simulink model "test_ffts"  (Simulink 6.2)
settings: Solver=ode45  StartTime=0.0  StopTime=300  RelTol=1e-3
undefined symbols (not defined in the file or in its folder): now
libraries: xbsIndex_r3 x1135, fft_library x1, simulink x1
(part 9 of 15)

== system test_ffts/r4_dit_fft/r4_dit_stage_3/quadplex_commutator ==
  a : Inport  Port=1  LatchInput=off
  b : Inport  Port=2  LatchInput=off
  c : Inport  Port=3  LatchInput=off
  d : Inport  Port=4  LatchInput=off
  sync_in : Inport  Port=5  LatchInput=off
  Terminator : Terminator
  biplex_commutator_01 : Subsystem  mask(Biplex Commutator){log2_size=1, n_bits=12, use_bram=off}
      mask prompts: log2_size "Log2 Block Size"; n_bits "Bit Width"; use_bram "Use BRAM"
      mask help: The biplex commutator commutes the first half of the BloBhi input "block" with the last half of the AloAhi input "block". A "block" is 2^log2_size consecutive samples (i.e. always a power of 2). sync_in precedes the first data input sample by one clock cycle. Overall latency from sync_in to sync_out is 2^(log2_size-1)+1.
      settings: AttributesFormatString=|
      | size = 2
      | delay slr
      mask Help:
      | <pre>
      | Description::
      | 
      | The biplex commutator commutes the first half of the BloBhi input "block"  with the last half
      | of the AloAhi input "block".  A "block" is 2^log2_size consecutive samples (i.e. always a
      | power of 2).
      | 
      | sync_in precedes the first data input sample by one clock cycle.
      | sync_out precedes the corresponding output sample by one clock cycle.
      | Overall latency from sync_in to sync_out is 2^(N-1)+1.
      | 
      | Mask Parameters::
      | 
      | Log 2 Block Size (log2_size): The base-2 logarithm of the length of one complete input block.
      | This MUST be an integer because the current implementation requires that
      | the input block size MUST be a power of 2.  (aka "N")
      | 
      | Bit Width (n_bits): Specifies the width of the real/imaginary components.
      | Width of each component is assumed equal.
      | 
      | Use BRAM (use_bram): Check this checkbox to implement the internal delays using BRAM.
      | If unchecked, the internal delays will be implemented using SLR16 elements.
      | </pre>
  biplex_commutator_23 : Subsystem  mask(Biplex Commutator){log2_size=1, n_bits=12, use_bram=off}
      mask prompts: log2_size "Log2 Block Size"; n_bits "Bit Width"; use_bram "Use BRAM"
      mask help: The biplex commutator commutes the first half of the BloBhi input "block" with the last half of the AloAhi input "block". A "block" is 2^log2_size consecutive samples (i.e. always a power of 2). sync_in precedes the first data input sample by one clock cycle. Overall latency from sync_in to sync_out is 2^(log2_size-1)+1.
      settings: AttributesFormatString=|
      | size = 2
      | delay slr
      mask Help:
      | <pre>
      | Description::
      | 
      | The biplex commutator commutes the first half of the BloBhi input "block"  with the last half
      | of the AloAhi input "block".  A "block" is 2^log2_size consecutive samples (i.e. always a
      | power of 2).
      | 
      | sync_in precedes the first data input sample by one clock cycle.
      | sync_out precedes the corresponding output sample by one clock cycle.
      | Overall latency from sync_in to sync_out is 2^(N-1)+1.
      | 
      | Mask Parameters::
      | 
      | Log 2 Block Size (log2_size): The base-2 logarithm of the length of one complete input block.
      | This MUST be an integer because the current implementation requires that
      | the input block size MUST be a power of 2.  (aka "N")
      | 
      | Bit Width (n_bits): Specifies the width of the real/imaginary components.
      | Width of each component is assumed equal.
      | 
      | Use BRAM (use_bram): Check this checkbox to implement the internal delays using BRAM.
      | If unchecked, the internal delays will be implemented using SLR16 elements.
      | </pre>
  biplex_commutator_ac : Subsystem  mask(Biplex Commutator){log2_size=2, n_bits=12, use_bram=off}
      mask prompts: log2_size "Log2 Block Size"; n_bits "Bit Width"; use_bram "Use BRAM"
      mask help: The biplex commutator commutes the first half of the BloBhi input "block" with the last half of the AloAhi input "block". A "block" is 2^log2_size consecutive samples (i.e. always a power of 2). sync_in precedes the first data input sample by one clock cycle. Overall latency from sync_in to sync_out is 2^(log2_size-1)+1.
      settings: AttributesFormatString=|
      | size = 4
      | delay slr
      mask Help:
      | <pre>
      | Description::
      | 
      | The biplex commutator commutes the first half of the BloBhi input "block"  with the last half
      | of the AloAhi input "block".  A "block" is 2^log2_size consecutive samples (i.e. always a
      | power of 2).
      | 
      | sync_in precedes the first data input sample by one clock cycle.
      | sync_out precedes the corresponding output sample by one clock cycle.
      | Overall latency from sync_in to sync_out is 2^(N-1)+1.
      | 
      | Mask Parameters::
      | 
      | Log 2 Block Size (log2_size): The base-2 logarithm of the length of one complete input block.
      | This MUST be an integer because the current implementation requires that
      | the input block size MUST be a power of 2.  (aka "N")
      | 
      | Bit Width (n_bits): Specifies the width of the real/imaginary components.
      | Width of each component is assumed equal.
      | 
      | Use BRAM (use_bram): Check this checkbox to implement the internal delays using BRAM.
      | If unchecked, the internal delays will be implemented using SLR16 elements.
      | </pre>
  biplex_commutator_bd : Subsystem  mask(Biplex Commutator){log2_size=2, n_bits=12, use_bram=off}
      mask prompts: log2_size "Log2 Block Size"; n_bits "Bit Width"; use_bram "Use BRAM"
      mask help: The biplex commutator commutes the first half of the BloBhi input "block" with the last half of the AloAhi input "block". A "block" is 2^log2_size consecutive samples (i.e. always a power of 2). sync_in precedes the first data input sample by one clock cycle. Overall latency from sync_in to sync_out is 2^(log2_size-1)+1.
      settings: AttributesFormatString=|
      | size = 4
      | delay slr
      mask Help:
      | <pre>
      | Description::
      | 
      | The biplex commutator commutes the first half of the BloBhi input "block"  with the last half
      | of the AloAhi input "block".  A "block" is 2^log2_size consecutive samples (i.e. always a
      | power of 2).
      | 
      | sync_in precedes the first data input sample by one clock cycle.
      | sync_out precedes the corresponding output sample by one clock cycle.
      | Overall latency from sync_in to sync_out is 2^(N-1)+1.
      | 
      | Mask Parameters::
      | 
      | Log 2 Block Size (log2_size): The base-2 logarithm of the length of one complete input block.
      | This MUST be an integer because the current implementation requires that
      | the input block size MUST be a power of 2.  (aka "N")
      | 
      | Bit Width (n_bits): Specifies the width of the real/imaginary components.
      | Width of each component is assumed equal.
      | 
      | Use BRAM (use_bram): Check this checkbox to implement the internal delays using BRAM.
      | If unchecked, the internal delays will be implemented using SLR16 elements.
      | </pre>
  abcd0 : Outport
  abcd1 : Outport  Port=2
  abcd2 : Outport  Port=3
  abcd3 : Outport  Port=4
  sync_out : Outport  Port=5
  wires:
  biplex_commutator_01/3(sync_out) -> Terminator/1
  biplex_commutator_23/3(sync_out) -> sync_out/1
  sync_in/1 -> biplex_commutator_bd/3(sync_in), biplex_commutator_ac/3(sync_in)
  d/1 -> biplex_commutator_bd/2(BloBhi)
  b/1 -> biplex_commutator_bd/1(AloAhi)
  c/1 -> biplex_commutator_ac/2(BloBhi)
  biplex_commutator_bd/3(sync_out) -> biplex_commutator_23/3(sync_in)
  biplex_commutator_bd/2(AhiBhi) -> biplex_commutator_23/2(BloBhi)
  biplex_commutator_ac/3(sync_out) -> biplex_commutator_01/3(sync_in)
  biplex_commutator_bd/1(AloBlo) -> biplex_commutator_01/2(BloBhi)
  biplex_commutator_ac/2(AhiBhi) -> biplex_commutator_23/1(AloAhi)
  biplex_commutator_23/2(AhiBhi) -> abcd3/1
  biplex_commutator_23/1(AloBlo) -> abcd2/1
  biplex_commutator_01/2(AhiBhi) -> abcd1/1
  biplex_commutator_01/1(AloBlo) -> abcd0/1
  a/1 -> biplex_commutator_ac/1(AloAhi)
  biplex_commutator_ac/1(AloBlo) -> biplex_commutator_01/1(AloAhi)

== system test_ffts/r4_dit_fft/r4_dit_stage_3/r4_butterfly ==
  a_in : Inport  Port=1  LatchInput=off
  b_in : Inport  Port=2  LatchInput=off
  c_in : Inport  Port=3  LatchInput=off
  d_in : Inport  Port=4  LatchInput=off
  sync_in : Inport  Port=5  LatchInput=off
  Terminator : Terminator
  butterfly0 : Subsystem  mask(Radix-2 Butterfly){n_bits=12, shift=0, quantization=Truncate, add_latency=1}
      mask prompts: n_bits "Bit Width In"; shift "Shift Bits"; add_latency "Adder Latency"
      mask help: The radix-2 butterfly produces a+b and a-b outputs for a and b inputs.
      settings: AttributesFormatString=shift 0
      mask Help:
      | <pre>
      | Description::
      | 
      | The radix-2 butterfly produces a+b and a-b outputs for a and b inputs.
      | The outputs are one bit wider than the inputs.
      | The output precision (i.e. the number of fractional bits) stays the same.
      | 
      | Mask Parameters::
      | 
      | Bit Width In (n_bits): Specifies the width of the real/imaginary components.
      | Width of each component is assumed equal.
      | 
      | Shift Bits (shift): Specifies how many bits to shift (down) by.  A positive value causes
      | the specified number of least significant bits to be dropped.  Usually zero or positive values
      | are used to permit or limit bit growth, but negative values can be used to induce bit growth.
      | 
      | Quantization (quantization): Specifies quantization handling (when shift bits > 0).
      | 
      | Adder Latency (add_latency): Latency to use for the underlying real adders.
      | </pre>
      mask StyleString: edit,edit,popup(Truncate|Round  (unbiased: +/- Inf)|Round  (unbiased: Even Values)),edit
  butterfly1 : Subsystem  mask(Radix-2 Butterfly){n_bits=12, shift=0, quantization=Truncate, add_latency=1}
      mask prompts: n_bits "Bit Width In"; shift "Shift Bits"; add_latency "Adder Latency"
      mask help: The radix-2 butterfly produces a+b and a-b outputs for a and b inputs.
      settings: AttributesFormatString=shift 0
      mask Help:
      | <pre>
      | Description::
      | 
      | The radix-2 butterfly produces a+b and a-b outputs for a and b inputs.
      | The outputs are one bit wider than the inputs.
      | The output precision (i.e. the number of fractional bits) stays the same.
      | 
      | Mask Parameters::
      | 
      | Bit Width In (n_bits): Specifies the width of the real/imaginary components.
      | Width of each component is assumed equal.
      | 
      | Shift Bits (shift): Specifies how many bits to shift (down) by.  A positive value causes
      | the specified number of least significant bits to be dropped.  Usually zero or positive values
      | are used to permit or limit bit growth, but negative values can be used to induce bit growth.
      | 
      | Quantization (quantization): Specifies quantization handling (when shift bits > 0).
      | 
      | Adder Latency (add_latency): Latency to use for the underlying real adders.
      | </pre>
      mask StyleString: edit,edit,popup(Truncate|Round  (unbiased: +/- Inf)|Round  (unbiased: Even Values)),edit
  butterfly2 : Subsystem  mask(Radix-2 Butterfly){n_bits=13, shift=0, quantization=Truncate, add_latency=1}
      mask prompts: n_bits "Bit Width In"; shift "Shift Bits"; add_latency "Adder Latency"
      mask help: The radix-2 butterfly produces a+b and a-b outputs for a and b inputs.
      settings: AttributesFormatString=shift 0
      mask Help:
      | <pre>
      | Description::
      | 
      | The radix-2 butterfly produces a+b and a-b outputs for a and b inputs.
      | The outputs are one bit wider than the inputs.
      | The output precision (i.e. the number of fractional bits) stays the same.
      | 
      | Mask Parameters::
      | 
      | Bit Width In (n_bits): Specifies the width of the real/imaginary components.
      | Width of each component is assumed equal.
      | 
      | Shift Bits (shift): Specifies how many bits to shift (down) by.  A positive value causes
      | the specified number of least significant bits to be dropped.  Usually zero or positive values
      | are used to permit or limit bit growth, but negative values can be used to induce bit growth.
      | 
      | Quantization (quantization): Specifies quantization handling (when shift bits > 0).
      | 
      | Adder Latency (add_latency): Latency to use for the underlying real adders.
      | </pre>
      mask StyleString: edit,edit,popup(Truncate|Round  (unbiased: +/- Inf)|Round  (unbiased: Even Values)),edit
  butterfly3j : Subsystem  mask(Radix-2 Butterfly with fixed -j twiddle (DIT, twiddle before butterfly)){n_bits=13, shift=0, quantization=Truncate, add_latency=1}
      mask prompts: n_bits "Bit Width In"; shift "Shift Bits"; add_latency "Adder Latency"
      mask help: The radix-2 butterfly with fixed DIT -j twiddle produces a-jb on the a+b output and a+jb on the a-b output for a and b inputs. It is intended for use within a radix-4 butterfly.
      settings: AttributesFormatString=shift 0
      mask Help:
      | <pre>
      | Description::
      | 
      | The radix-2 butterfly with fixed DIT -j twiddle produces a-jb on the a+b output
      | and a+jb on the a-b output for a and b inputs.
      | 
      | It is intended for use within a radix-4 butterfly.
      | 
      | The outputs are one bit wider than the inputs.
      | The output precision (i.e. the number of fractional bits) stays the same.
      | 
      | Mask Parameters::
      | 
      | Bit Width In (n_bits): Specifies the width of the real/imaginary components.
      | Width of each component is assumed equal.
      | 
      | Shift Bits (shift): Specifies how many bits to shift (down) by.  A positive value causes
      | the specified number of least significant bits to be dropped.  Usually zero or positive values
      | are used to permit or limit bit growth, but negative values can be used to induce bit growth.
      | 
      | Quantization (quantization): Specifies quantization handling (when shift bits > 0).
      | 
      | Adder Latency (add_latency): Latency to use for the underlying real adders.
      | </pre>
      mask StyleString: edit,edit,popup(Truncate|Round  (unbiased: +/- Inf)|Round  (unbiased: Even Values)),edit
  a_out : Outport
  b_out : Outport  Port=2
  c_out : Outport  Port=3
  d_out : Outport  Port=4
  sync_out : Outport  Port=5
  wires:
  butterfly2/3(sync_out) -> Terminator/1
  butterfly3j/3(sync_out) -> sync_out/1
  sync_in/1 -> butterfly0/3(sync_in), butterfly1/3(sync_in)
  butterfly3j/2(a-b) -> d_out/1
  butterfly3j/1(a+b) -> c_out/1
  butterfly2/2(a-b) -> b_out/1
  butterfly2/1(a+b) -> a_out/1
  b_in/1 -> butterfly1/1(a)
  d_in/1 -> butterfly1/2(b)
  c_in/1 -> butterfly0/2(b)
  a_in/1 -> butterfly0/1(a)
  butterfly1/1(a+b) -> butterfly2/2(b)
  butterfly0/2(a-b) -> butterfly3j/1(a)
  butterfly0/3(sync_out) -> butterfly2/3(sync_in)
  butterfly1/3(sync_out) -> butterfly3j/3(sync_in)
  butterfly1/2(a-b) -> butterfly3j/2(b)
  butterfly0/1(a+b) -> butterfly2/1(a)

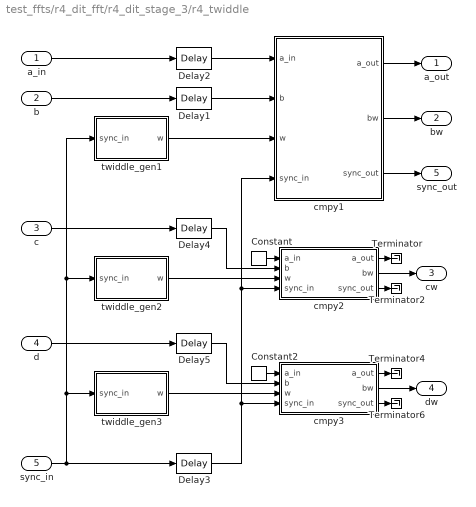
== system test_ffts/r4_dit_fft/r4_dit_stage_3/r4_twiddle ==
  a_in : Inport  Port=1  LatchInput=off
  b : Inport  Port=2  LatchInput=off
  c : Inport  Port=3  LatchInput=off
  d : Inport  Port=4  LatchInput=off
  sync_in : Inport  Port=5  LatchInput=off
  Constant : xbsIndex_r3/Constant  const=0  equ=P=C  arith_type=Unsigned  n_bits=1  bin_pt=0  opselect=C  inp2=PCIN>>17  opr=+  inp1=P  carry=CIN  iostate=0  explicit_period=on  period=1  dbl_ovrd=off
  Constant2 : xbsIndex_r3/Constant  const=0  equ=P=C  arith_type=Unsigned  n_bits=1  bin_pt=0  opselect=C  inp2=PCIN>>17  opr=+  inp1=P  carry=CIN  iostate=0  explicit_period=on  period=1  dbl_ovrd=off
  Delay{1..5} (5 alike) : xbsIndex_r3/Delay  latency=1  reg_retiming=off  explicit_period=off  period=1  en=off  accept_only_valid=off  init_zero=on  dbl_ovrd=off  show_param=off
      settings: xl_area=[0, 0, 0, 0, 0, 0, 0]
  Terminator{,2,4,6} (4 alike) : Terminator
  cmpy1 : Subsystem  mask(Complex Multiplier (4 real multipliers)){n_bits_b=12, bin_pt_b=11, n_bits_w=9, bin_pt_w=7, n_bits_bw=12, bin_pt_bw=11, quantization=Round  (unbiased: Even Values), overflow=Wrap, mult_latency=3, add_latency=1}
      mask prompts: n_bits_b "Number of Bits B"; bin_pt_b "Binary Point B"; n_bits_w "Number of Bits W"; bin_pt_w "Binary Point W"; n_bits_bw "Number of Bits BW"; bin_pt_bw "Binary Point BW"; mult_latency "Multiplier Latency"; add_latency "Adder Latency"
      mask help: This block multiplies two complex numbers using 4 real multipliers and 2 real adders. Pass-through paths are provided for another complex number and a sync signal. These pass through paths provide delay that matches the latency of the complex multiply operation.
      settings: AttributesFormatString=|
      | 12_11 * 9_7 ==> 12_11
      | round even, wrap
      | 3 mults
      mask Help:
      | <pre>
      | Description::
      | 
      | This block multiplies two complex numbers using 4 real multipliers and 2 real adders.
      | Pass-through paths are provided for another complex number and a sync signal.
      | These paths provide delay that matches the latency of the complex multiply operation.
      | 
      | a_in is passed through to a_out.
      | b and w complex inputs are multiplied and their product appears on the bw output.
      | sync_in is passed through to sync_out.
      | 
      | Mask Parameters::
      | 
      | Number of Bits B (n_bits_b): Specifies the width of the real/imaginary
      | components of input b.  Assumed equal for both components.
      | 
      | Binary Point B (bin_pt_b): Specifies the binary point point position of the
      | real/imaginary components of input b.  Assumed equal for both components.
      | 
      | Number of Bits W (n_bits_w): Specifies the width of the real/imaginary
      | components of input w.  Assumed equal for both components.
      | 
      | Binary Point W (bin_pt_w): Specifies the binary point point position of the
      | real/imaginary components of input w.  Assumed equal for both components.
      | 
      | Number of Bits BW (n_bits_bw): Specifies the width of the real/imaginary
      | components of output bw.  Assumed equal for both components.
      | 
      | Binary Point BW (bin_pt_bw): Specifies the binary point point position of the
      | real/imaginary components of output bw.  Assumed equal for both components.
      | 
      | Quantization (quantization): Specifies quantization handling.
      | 
      | Overflow (overflow): Specifies overflow handling.
      | 
      | Multiplier Latency (mult_latency): Latency to use for the underlying real multipliers.
      | 
      | Adder Latency (add_latency): Latency to use for the underlying real adders.
      | </pre>
      mask StyleString: edit,edit,edit,edit,edit,edit,popup(Truncate|Round  (unbiased: +/- Inf)|Round  (unbiased: Even Values)),popup(Wrap|Saturate|Error),edit,edit
  cmpy2 : Subsystem  mask(Complex Multiplier (4 real multipliers)){n_bits_b=12, bin_pt_b=11, n_bits_w=9, bin_pt_w=7, n_bits_bw=12, bin_pt_bw=11, quantization=Round  (unbiased: Even Values), overflow=Wrap, mult_latency=3, add_latency=1}
      mask prompts: n_bits_b "Number of Bits B"; bin_pt_b "Binary Point B"; n_bits_w "Number of Bits W"; bin_pt_w "Binary Point W"; n_bits_bw "Number of Bits BW"; bin_pt_bw "Binary Point BW"; mult_latency "Multiplier Latency"; add_latency "Adder Latency"
      mask help: This block multiplies two complex numbers using 4 real multipliers and 2 real adders. Pass-through paths are provided for another complex number and a sync signal. These pass through paths provide delay that matches the latency of the complex multiply operation.
      settings: AttributesFormatString=|
      | 12_11 * 9_7 ==> 12_11
      | round even, wrap
      | 3 mults
      mask Help:
      | <pre>
      | Description::
      | 
      | This block multiplies two complex numbers using 4 real multipliers and 2 real adders.
      | Pass-through paths are provided for another complex number and a sync signal.
      | These paths provide delay that matches the latency of the complex multiply operation.
      | 
      | a_in is passed through to a_out.
      | b and w complex inputs are multiplied and their product appears on the bw output.
      | sync_in is passed through to sync_out.
      | 
      | Mask Parameters::
      | 
      | Number of Bits B (n_bits_b): Specifies the width of the real/imaginary
      | components of input b.  Assumed equal for both components.
      | 
      | Binary Point B (bin_pt_b): Specifies the binary point point position of the
      | real/imaginary components of input b.  Assumed equal for both components.
      | 
      | Number of Bits W (n_bits_w): Specifies the width of the real/imaginary
      | components of input w.  Assumed equal for both components.
      | 
      | Binary Point W (bin_pt_w): Specifies the binary point point position of the
      | real/imaginary components of input w.  Assumed equal for both components.
      | 
      | Number of Bits BW (n_bits_bw): Specifies the width of the real/imaginary
      | components of output bw.  Assumed equal for both components.
      | 
      | Binary Point BW (bin_pt_bw): Specifies the binary point point position of the
      | real/imaginary components of output bw.  Assumed equal for both components.
      | 
      | Quantization (quantization): Specifies quantization handling.
      | 
      | Overflow (overflow): Specifies overflow handling.
      | 
      | Multiplier Latency (mult_latency): Latency to use for the underlying real multipliers.
      | 
      | Adder Latency (add_latency): Latency to use for the underlying real adders.
      | </pre>
      mask StyleString: edit,edit,edit,edit,edit,edit,popup(Truncate|Round  (unbiased: +/- Inf)|Round  (unbiased: Even Values)),popup(Wrap|Saturate|Error),edit,edit
  cmpy3 : Subsystem  mask(Complex Multiplier (4 real multipliers)){n_bits_b=12, bin_pt_b=11, n_bits_w=9, bin_pt_w=7, n_bits_bw=12, bin_pt_bw=11, quantization=Round  (unbiased: Even Values), overflow=Wrap, mult_latency=3, add_latency=1}
      mask prompts: n_bits_b "Number of Bits B"; bin_pt_b "Binary Point B"; n_bits_w "Number of Bits W"; bin_pt_w "Binary Point W"; n_bits_bw "Number of Bits BW"; bin_pt_bw "Binary Point BW"; mult_latency "Multiplier Latency"; add_latency "Adder Latency"
      mask help: This block multiplies two complex numbers using 4 real multipliers and 2 real adders. Pass-through paths are provided for another complex number and a sync signal. These pass through paths provide delay that matches the latency of the complex multiply operation.
      settings: AttributesFormatString=|
      | 12_11 * 9_7 ==> 12_11
      | round even, wrap
      | 3 mults
      mask Help:
      | <pre>
      | Description::
      | 
      | This block multiplies two complex numbers using 4 real multipliers and 2 real adders.
      | Pass-through paths are provided for another complex number and a sync signal.
      | These paths provide delay that matches the latency of the complex multiply operation.
      | 
      | a_in is passed through to a_out.
      | b and w complex inputs are multiplied and their product appears on the bw output.
      | sync_in is passed through to sync_out.
      | 
      | Mask Parameters::
      | 
      | Number of Bits B (n_bits_b): Specifies the width of the real/imaginary
      | components of input b.  Assumed equal for both components.
      | 
      | Binary Point B (bin_pt_b): Specifies the binary point point position of the
      | real/imaginary components of input b.  Assumed equal for both components.
      | 
      | Number of Bits W (n_bits_w): Specifies the width of the real/imaginary
      | components of input w.  Assumed equal for both components.
      | 
      | Binary Point W (bin_pt_w): Specifies the binary point point position of the
      | real/imaginary components of input w.  Assumed equal for both components.
      | 
      | Number of Bits BW (n_bits_bw): Specifies the width of the real/imaginary
      | components of output bw.  Assumed equal for both components.
      | 
      | Binary Point BW (bin_pt_bw): Specifies the binary point point position of the
      | real/imaginary components of output bw.  Assumed equal for both components.
      | 
      | Quantization (quantization): Specifies quantization handling.
      | 
      | Overflow (overflow): Specifies overflow handling.
      | 
      | Multiplier Latency (mult_latency): Latency to use for the underlying real multipliers.
      | 
      | Adder Latency (add_latency): Latency to use for the underlying real adders.
      | </pre>
      mask StyleString: edit,edit,edit,edit,edit,edit,popup(Truncate|Round  (unbiased: +/- Inf)|Round  (unbiased: Even Values)),popup(Wrap|Saturate|Error),edit,edit
  twiddle_gen1 : Subsystem  mask(Radix-R Twiddle Coefficient Generator (complex storage)){n_stages=3, radix=4, cur_stage=3, branch=1, decimation=Time, n_bits_w=9, bin_pt_w=7, use_bram=off}
      mask prompts: n_stages "Total Stages"; cur_stage "Current Stage"; decimation "Decimation Mode"; n_bits_w "Number of Bits"; bin_pt_w "Binary Point"; use_bram "Use BRAM"
      mask help: A radix-R twiddle coefficient generator using complex storage. Generates twiddle factors for Decimation in Time (i.e. twiddles before butterflies) or Decimation in Frequency (i.e. twiddles after butterflies) Fast Fourier Transforms of arbitrary-but-fixed radix. Radix must be a power of 2. Regardless of the decimation mode, the FFT is assumed to have inputs in normal order and outputs in bit-reversed order.
      settings: AttributesFormatString=|
      | depth 16
      | twiddle dist
      mask Help:
      | <pre>
      | Description::
      | 
      | A radix-R twiddle coefficient generator using complex storage.
      | 
      | Generates twiddle factors for Decimation in Time (i.e. twiddles before butterflies)
      | or Decimation in Frequency (i.e. twiddles after butterflies) Fast Fourier Transforms
      | of arbitrary-but-fixed radix.  Radix must be a power of 2.
      | 
      | Regardless of the decimation mode, the FFT is assumed to have inputs normally
      | ordered and outputs in bit-reversed order.
      | 
      | Complex storage means that the real and imaginary components are stored in
      | the same memory element.  This is generally fine, but if the combined width of
      | the real and imaginary components is greater than 18 and BRAM is being used
      | for the underlying storage, then the multiplier(s) adjacent to the BRAM(s) will
      | not be usable.  If that is a problem for your design, consider using the
      | "Radix-R Twiddle Coefficient Generator (real/imag storage)" block.
      | 
      | Mask Parameters::
      | 
      | Total Stages (n_stages):  The number of total stages in the FFT.
      | 
      | Radix (radix): The radix of the FFT.  The FFT will have radix^n_stages points.
      | 
      | Current Stage (cur_stage):  The number of the current stage for which this block should
      | generate twiddle coefficients.  Valid values are 3 through n_stages, inclusive.  Note that
      | stages are counted from 1 to n_stages for DIT (i.e. cur_stage==1 for the first stage) and
      | n_stages to 1 for DIF (i.e. cur_stage==1 for the last stage).
      | 
      | Branch (branch): The butterfly branch associated with this twiddle generator.
      | Valid values are 1 through radix-1, inclusive.
      | 
      | Decimation Mode (decimation): The decimation mode of the FFT.
      | 
      | Number of Bits (n_bits_w): Specifies the width of the real/imaginary components.
      | Assumed equal for both components.  This block outputs UFix_(2*n_bits_w)_0.
      | 
      | Use BRAM (use_bram): Check this checkbox to store twiddle coefficients in BRAM.
      | If unchecked, the coefficients will be sored in distributed memory (i.e. slices).
      | </pre>
      mask StyleString: edit,edit,edit,edit,popup(Time|Frequency),edit,edit,checkbox
  twiddle_gen2 : Subsystem  mask(Radix-R Twiddle Coefficient Generator (complex storage)){n_stages=3, radix=4, cur_stage=3, branch=2, decimation=Time, n_bits_w=9, bin_pt_w=7, use_bram=off}
      mask prompts: n_stages "Total Stages"; cur_stage "Current Stage"; decimation "Decimation Mode"; n_bits_w "Number of Bits"; bin_pt_w "Binary Point"; use_bram "Use BRAM"
      mask help: A radix-R twiddle coefficient generator using complex storage. Generates twiddle factors for Decimation in Time (i.e. twiddles before butterflies) or Decimation in Frequency (i.e. twiddles after butterflies) Fast Fourier Transforms of arbitrary-but-fixed radix. Radix must be a power of 2. Regardless of the decimation mode, the FFT is assumed to have inputs in normal order and outputs in bit-reversed order.
      settings: AttributesFormatString=|
      | depth 16
      | twiddle dist
      mask Help:
      | <pre>
      | Description::
      | 
      | A radix-R twiddle coefficient generator using complex storage.
      | 
      | Generates twiddle factors for Decimation in Time (i.e. twiddles before butterflies)
      | or Decimation in Frequency (i.e. twiddles after butterflies) Fast Fourier Transforms
      | of arbitrary-but-fixed radix.  Radix must be a power of 2.
      | 
      | Regardless of the decimation mode, the FFT is assumed to have inputs normally
      | ordered and outputs in bit-reversed order.
      | 
      | Complex storage means that the real and imaginary components are stored in
      | the same memory element.  This is generally fine, but if the combined width of
      | the real and imaginary components is greater than 18 and BRAM is being used
      | for the underlying storage, then the multiplier(s) adjacent to the BRAM(s) will
      | not be usable.  If that is a problem for your design, consider using the
      | "Radix-R Twiddle Coefficient Generator (real/imag storage)" block.
      | 
      | Mask Parameters::
      | 
      | Total Stages (n_stages):  The number of total stages in the FFT.
      | 
      | Radix (radix): The radix of the FFT.  The FFT will have radix^n_stages points.
      | 
      | Current Stage (cur_stage):  The number of the current stage for which this block should
      | generate twiddle coefficients.  Valid values are 3 through n_stages, inclusive.  Note that
      | stages are counted from 1 to n_stages for DIT (i.e. cur_stage==1 for the first stage) and
      | n_stages to 1 for DIF (i.e. cur_stage==1 for the last stage).
      | 
      | Branch (branch): The butterfly branch associated with this twiddle generator.
      | Valid values are 1 through radix-1, inclusive.
      | 
      | Decimation Mode (decimation): The decimation mode of the FFT.
      | 
      | Number of Bits (n_bits_w): Specifies the width of the real/imaginary components.
      | Assumed equal for both components.  This block outputs UFix_(2*n_bits_w)_0.
      | 
      | Use BRAM (use_bram): Check this checkbox to store twiddle coefficients in BRAM.
      | If unchecked, the coefficients will be sored in distributed memory (i.e. slices).
      | </pre>
      mask StyleString: edit,edit,edit,edit,popup(Time|Frequency),edit,edit,checkbox
  twiddle_gen3 : Subsystem  mask(Radix-R Twiddle Coefficient Generator (complex storage)){n_stages=3, radix=4, cur_stage=3, branch=3, decimation=Time, n_bits_w=9, bin_pt_w=7, use_bram=off}
      mask prompts: n_stages "Total Stages"; cur_stage "Current Stage"; decimation "Decimation Mode"; n_bits_w "Number of Bits"; bin_pt_w "Binary Point"; use_bram "Use BRAM"
      mask help: A radix-R twiddle coefficient generator using complex storage. Generates twiddle factors for Decimation in Time (i.e. twiddles before butterflies) or Decimation in Frequency (i.e. twiddles after butterflies) Fast Fourier Transforms of arbitrary-but-fixed radix. Radix must be a power of 2. Regardless of the decimation mode, the FFT is assumed to have inputs in normal order and outputs in bit-reversed order.
      settings: AttributesFormatString=|
      | depth 16
      | twiddle dist
      mask Help:
      | <pre>
      | Description::
      | 
      | A radix-R twiddle coefficient generator using complex storage.
      | 
      | Generates twiddle factors for Decimation in Time (i.e. twiddles before butterflies)
      | or Decimation in Frequency (i.e. twiddles after butterflies) Fast Fourier Transforms
      | of arbitrary-but-fixed radix.  Radix must be a power of 2.
      | 
      | Regardless of the decimation mode, the FFT is assumed to have inputs normally
      | ordered and outputs in bit-reversed order.
      | 
      | Complex storage means that the real and imaginary components are stored in
      | the same memory element.  This is generally fine, but if the combined width of
      | the real and imaginary components is greater than 18 and BRAM is being used
      | for the underlying storage, then the multiplier(s) adjacent to the BRAM(s) will
      | not be usable.  If that is a problem for your design, consider using the
      | "Radix-R Twiddle Coefficient Generator (real/imag storage)" block.
      | 
      | Mask Parameters::
      | 
      | Total Stages (n_stages):  The number of total stages in the FFT.
      | 
      | Radix (radix): The radix of the FFT.  The FFT will have radix^n_stages points.
      | 
      | Current Stage (cur_stage):  The number of the current stage for which this block should
      | generate twiddle coefficients.  Valid values are 3 through n_stages, inclusive.  Note that
      | stages are counted from 1 to n_stages for DIT (i.e. cur_stage==1 for the first stage) and
      | n_stages to 1 for DIF (i.e. cur_stage==1 for the last stage).
      | 
      | Branch (branch): The butterfly branch associated with this twiddle generator.
      | Valid values are 1 through radix-1, inclusive.
      | 
      | Decimation Mode (decimation): The decimation mode of the FFT.
      | 
      | Number of Bits (n_bits_w): Specifies the width of the real/imaginary components.
      | Assumed equal for both components.  This block outputs UFix_(2*n_bits_w)_0.
      | 
      | Use BRAM (use_bram): Check this checkbox to store twiddle coefficients in BRAM.
      | If unchecked, the coefficients will be sored in distributed memory (i.e. slices).
      | </pre>
      mask StyleString: edit,edit,edit,edit,popup(Time|Frequency),edit,edit,checkbox
  a_out : Outport
  bw : Outport  Port=2
  cw : Outport  Port=3
  dw : Outport  Port=4
  sync_out : Outport  Port=5
  wires:
  Delay3/1 -> cmpy2/4(sync_in), cmpy1/4(sync_in), cmpy3/4(sync_in)
  cmpy3/3(sync_out) -> Terminator6/1
  cmpy3/1(a_out) -> Terminator4/1
  Constant2/1 -> cmpy3/1(a_in)
  cmpy2/3(sync_out) -> Terminator2/1
  cmpy2/1(a_out) -> Terminator/1
  Constant/1 -> cmpy2/1(a_in)
  Delay5/1 -> cmpy3/2(b)
  d/1 -> Delay5/1
  Delay4/1 -> cmpy2/2(b)
  c/1 -> Delay4/1
  twiddle_gen3/1(w) -> cmpy3/3(w)
  twiddle_gen2/1(w) -> cmpy2/3(w)
  cmpy3/2(bw) -> dw/1
  cmpy2/2(bw) -> cw/1
  sync_in/1 -> twiddle_gen3/1(sync_in), twiddle_gen2/1(sync_in), twiddle_gen1/1(sync_in), Delay3/1
  b/1 -> Delay1/1
  a_in/1 -> Delay2/1
  Delay2/1 -> cmpy1/1(a_in)
  cmpy1/1(a_out) -> a_out/1
  Delay1/1 -> cmpy1/2(b)
  cmpy1/2(bw) -> bw/1
  twiddle_gen1/1(w) -> cmpy1/3(w)
  cmpy1/3(sync_out) -> sync_out/1

== system test_ffts/r2_dit_fft/biplex_commutator/delay_b/c_to_ri ==
  c : Inport  Port=1  LatchInput=off
  force_im : xbsIndex_r3/Reinterpret  force_arith_type=on  arith_type="Signed  (2's comp)"  force_bin_pt=on  bin_pt=0  force_valid=on
  force_re : xbsIndex_r3/Reinterpret  force_arith_type=on  arith_type="Signed  (2's comp)"  force_bin_pt=on  bin_pt=0  force_valid=on
  slice_im : xbsIndex_r3/Slice  mode=Lower Bit Location + Width  nbits=14  bit1=0  base1=MSB of Input  bit0=0  base0=LSB of Input  boolean_output=off  explicit_period=off  period=1  dbl_ovrd=off
  slice_re : xbsIndex_r3/Slice  mode=Upper Bit Location + Width  nbits=14  bit1=0  base1=MSB of Input  bit0=0  base0=LSB of Input  boolean_output=off  explicit_period=off  period=1  dbl_ovrd=off
  re : Outport
  im : Outport  Port=2
  wires:
  slice_re/1 -> force_re/1
  slice_im/1 -> force_im/1
  force_re/1 -> re/1
  force_im/1 -> im/1
  c/1 -> slice_re/1, slice_im/1

== system test_ffts/r2_dit_fft/biplex_commutator/delay_b/delay_im ==
  in : Inport  Port=1  LatchInput=off
  Constant : xbsIndex_r3/Constant  const=1  equ=P=C  arith_type=Boolean  n_bits=1  bin_pt=0  opselect=C  inp2=PCIN>>17  opr=+  inp1=P  carry=CIN  iostate=0  explicit_period=on  period=1  dbl_ovrd=off
  Counter : xbsIndex_r3/Counter  cnt_type=Count Limited  n_bits=5  bin_pt=0  arith_type=Unsigned  start_count=0  cnt_to=30  cnt_by_val=1  operation=Up  explicit_period=off  period=1  load_pin=off  rst=off  en=off  dbl_ovrd=off  show_param=off  use_rpm=on  gen_core=off
      settings: xl_area=[0, 0, 0, 0, 0, 0, 0]
  bram : xbsIndex_r3/Single Port RAM  depth=32  initVector=0  write_mode=Read Before Write  latency=1  init_zero=on  explicit_period=off  period=1  rst=off  init_reg=0  en=off  dbl_ovrd=off  show_param=off  distributed_mem=off  use_rpm=off  gen_core=off
      settings: xl_area=[0, 0, 0, 0, 0, 0, 0]
  out : Outport
  wires:
  Constant/1 -> bram/3
  in/1 -> bram/2
  bram/1 -> out/1
  Counter/1 -> bram/1

== system test_ffts/r2_dit_fft/biplex_commutator/delay_b/delay_re ==
  in : Inport  Port=1  LatchInput=off
  Constant : xbsIndex_r3/Constant  const=1  equ=P=C  arith_type=Boolean  n_bits=1  bin_pt=0  opselect=C  inp2=PCIN>>17  opr=+  inp1=P  carry=CIN  iostate=0  explicit_period=on  period=1  dbl_ovrd=off
  Counter : xbsIndex_r3/Counter  cnt_type=Count Limited  n_bits=5  bin_pt=0  arith_type=Unsigned  start_count=0  cnt_to=30  cnt_by_val=1  operation=Up  explicit_period=off  period=1  load_pin=off  rst=off  en=off  dbl_ovrd=off  show_param=off  use_rpm=on  gen_core=off
      settings: xl_area=[0, 0, 0, 0, 0, 0, 0]
  bram : xbsIndex_r3/Single Port RAM  depth=32  initVector=0  write_mode=Read Before Write  latency=1  init_zero=on  explicit_period=off  period=1  rst=off  init_reg=0  en=off  dbl_ovrd=off  show_param=off  distributed_mem=off  use_rpm=off  gen_core=off
      settings: xl_area=[0, 0, 0, 0, 0, 0, 0]
  out : Outport
  wires:
  Constant/1 -> bram/3
  in/1 -> bram/2
  bram/1 -> out/1
  Counter/1 -> bram/1

== system test_ffts/r2_dit_fft/biplex_commutator/delay_b/ri_to_c ==
  re : Inport  Port=1  LatchInput=off
  im : Inport  Port=2  LatchInput=off
  concat : xbsIndex_r3/Concat  num_inputs=2  explicit_period=off  period=1  dbl_ovrd=off
  force_im : xbsIndex_r3/Reinterpret  force_arith_type=on  arith_type=Unsigned  force_bin_pt=on  bin_pt=0  force_valid=on
  force_re : xbsIndex_r3/Reinterpret  force_arith_type=on  arith_type=Unsigned  force_bin_pt=on  bin_pt=0  force_valid=on
  c : Outport
  wires:
  force_re/1 -> concat/1
  force_im/1 -> concat/2
  re/1 -> force_re/1
  concat/1 -> c/1
  im/1 -> force_im/1

== system test_ffts/r2_dit_fft/biplex_commutator/delay_lo/c_to_ri ==
  c : Inport  Port=1  LatchInput=off
  force_im : xbsIndex_r3/Reinterpret  force_arith_type=on  arith_type="Signed  (2's comp)"  force_bin_pt=on  bin_pt=0  force_valid=on
  force_re : xbsIndex_r3/Reinterpret  force_arith_type=on  arith_type="Signed  (2's comp)"  force_bin_pt=on  bin_pt=0  force_valid=on
  slice_im : xbsIndex_r3/Slice  mode=Lower Bit Location + Width  nbits=14  bit1=0  base1=MSB of Input  bit0=0  base0=LSB of Input  boolean_output=off  explicit_period=off  period=1  dbl_ovrd=off
  slice_re : xbsIndex_r3/Slice  mode=Upper Bit Location + Width  nbits=14  bit1=0  base1=MSB of Input  bit0=0  base0=LSB of Input  boolean_output=off  explicit_period=off  period=1  dbl_ovrd=off
  re : Outport
  im : Outport  Port=2
  wires:
  slice_re/1 -> force_re/1
  slice_im/1 -> force_im/1
  force_re/1 -> re/1
  force_im/1 -> im/1
  c/1 -> slice_re/1, slice_im/1

== system test_ffts/r2_dit_fft/biplex_commutator/delay_lo/delay_im ==
  in : Inport  Port=1  LatchInput=off
  Constant : xbsIndex_r3/Constant  const=1  equ=P=C  arith_type=Boolean  n_bits=1  bin_pt=0  opselect=C  inp2=PCIN>>17  opr=+  inp1=P  carry=CIN  iostate=0  explicit_period=on  period=1  dbl_ovrd=off
  Counter : xbsIndex_r3/Counter  cnt_type=Count Limited  n_bits=5  bin_pt=0  arith_type=Unsigned  start_count=0  cnt_to=30  cnt_by_val=1  operation=Up  explicit_period=off  period=1  load_pin=off  rst=off  en=off  dbl_ovrd=off  show_param=off  use_rpm=on  gen_core=off
      settings: xl_area=[0, 0, 0, 0, 0, 0, 0]
  bram : xbsIndex_r3/Single Port RAM  depth=32  initVector=0  write_mode=Read Before Write  latency=1  init_zero=on  explicit_period=off  period=1  rst=off  init_reg=0  en=off  dbl_ovrd=off  show_param=off  distributed_mem=off  use_rpm=off  gen_core=off
      settings: xl_area=[0, 0, 0, 0, 0, 0, 0]
  out : Outport
  wires:
  Constant/1 -> bram/3
  in/1 -> bram/2
  bram/1 -> out/1
  Counter/1 -> bram/1

== system test_ffts/r2_dit_fft/biplex_commutator/delay_lo/delay_re ==
  in : Inport  Port=1  LatchInput=off
  Constant : xbsIndex_r3/Constant  const=1  equ=P=C  arith_type=Boolean  n_bits=1  bin_pt=0  opselect=C  inp2=PCIN>>17  opr=+  inp1=P  carry=CIN  iostate=0  explicit_period=on  period=1  dbl_ovrd=off
  Counter : xbsIndex_r3/Counter  cnt_type=Count Limited  n_bits=5  bin_pt=0  arith_type=Unsigned  start_count=0  cnt_to=30  cnt_by_val=1  operation=Up  explicit_period=off  period=1  load_pin=off  rst=off  en=off  dbl_ovrd=off  show_param=off  use_rpm=on  gen_core=off
      settings: xl_area=[0, 0, 0, 0, 0, 0, 0]
  bram : xbsIndex_r3/Single Port RAM  depth=32  initVector=0  write_mode=Read Before Write  latency=1  init_zero=on  explicit_period=off  period=1  rst=off  init_reg=0  en=off  dbl_ovrd=off  show_param=off  distributed_mem=off  use_rpm=off  gen_core=off
      settings: xl_area=[0, 0, 0, 0, 0, 0, 0]
  out : Outport
  wires:
  Constant/1 -> bram/3
  in/1 -> bram/2
  bram/1 -> out/1
  Counter/1 -> bram/1

== system test_ffts/r2_dit_fft/biplex_commutator/delay_lo/ri_to_c ==
  re : Inport  Port=1  LatchInput=off
  im : Inport  Port=2  LatchInput=off
  concat : xbsIndex_r3/Concat  num_inputs=2  explicit_period=off  period=1  dbl_ovrd=off
  force_im : xbsIndex_r3/Reinterpret  force_arith_type=on  arith_type=Unsigned  force_bin_pt=on  bin_pt=0  force_valid=on
  force_re : xbsIndex_r3/Reinterpret  force_arith_type=on  arith_type=Unsigned  force_bin_pt=on  bin_pt=0  force_valid=on
  c : Outport
  wires:
  force_re/1 -> concat/1
  force_im/1 -> concat/2
  re/1 -> force_re/1
  concat/1 -> c/1
  im/1 -> force_im/1

== system test_ffts/r2_dit_fft/r2_dit_stage_1/biplex_commutator/delay_b ==
  in : Inport  Port=1  LatchInput=off
  slr : xbsIndex_r3/Delay  latency=32  reg_retiming=off  explicit_period=off  period=1  en=off  accept_only_valid=off  init_zero=on  dbl_ovrd=off  show_param=off
      settings: xl_area=[0, 0, 0, 0, 0, 0, 0]
  out : Outport
  wires:
  slr/1 -> out/1
  in/1 -> slr/1

== system test_ffts/r2_dit_fft/r2_dit_stage_1/biplex_commutator/delay_lo ==
  in : Inport  Port=1  LatchInput=off
  slr : xbsIndex_r3/Delay  latency=32  reg_retiming=off  explicit_period=off  period=1  en=off  accept_only_valid=off  init_zero=on  dbl_ovrd=off  show_param=off
      settings: xl_area=[0, 0, 0, 0, 0, 0, 0]
  out : Outport
  wires:
  slr/1 -> out/1
  in/1 -> slr/1

== system test_ffts/r2_dit_fft/r2_dit_stage_1/r2_butterfly/c_to_ri ==
  c : Inport  Port=1  LatchInput=off
  force_im : xbsIndex_r3/Reinterpret  force_arith_type=on  arith_type="Signed  (2's comp)"  force_bin_pt=on  bin_pt=0  force_valid=on
  force_re : xbsIndex_r3/Reinterpret  force_arith_type=on  arith_type="Signed  (2's comp)"  force_bin_pt=on  bin_pt=0  force_valid=on
  slice_im : xbsIndex_r3/Slice  mode=Lower Bit Location + Width  nbits=8  bit1=0  base1=MSB of Input  bit0=0  base0=LSB of Input  boolean_output=off  explicit_period=off  period=1  dbl_ovrd=off
  slice_re : xbsIndex_r3/Slice  mode=Upper Bit Location + Width  nbits=8  bit1=0  base1=MSB of Input  bit0=0  base0=LSB of Input  boolean_output=off  explicit_period=off  period=1  dbl_ovrd=off
  re : Outport
  im : Outport  Port=2
  wires:
  slice_re/1 -> force_re/1
  slice_im/1 -> force_im/1
  force_re/1 -> re/1
  force_im/1 -> im/1
  c/1 -> slice_re/1, slice_im/1

== system test_ffts/r2_dit_fft/r2_dit_stage_1/r2_butterfly/c_to_ri1 ==
  c : Inport  Port=1  LatchInput=off
  force_im : xbsIndex_r3/Reinterpret  force_arith_type=on  arith_type="Signed  (2's comp)"  force_bin_pt=on  bin_pt=0  force_valid=on
  force_re : xbsIndex_r3/Reinterpret  force_arith_type=on  arith_type="Signed  (2's comp)"  force_bin_pt=on  bin_pt=0  force_valid=on
  slice_im : xbsIndex_r3/Slice  mode=Lower Bit Location + Width  nbits=8  bit1=0  base1=MSB of Input  bit0=0  base0=LSB of Input  boolean_output=off  explicit_period=off  period=1  dbl_ovrd=off
  slice_re : xbsIndex_r3/Slice  mode=Upper Bit Location + Width  nbits=8  bit1=0  base1=MSB of Input  bit0=0  base0=LSB of Input  boolean_output=off  explicit_period=off  period=1  dbl_ovrd=off
  re : Outport
  im : Outport  Port=2
  wires:
  slice_re/1 -> force_re/1
  slice_im/1 -> force_im/1
  force_re/1 -> re/1
  force_im/1 -> im/1
  c/1 -> slice_re/1, slice_im/1

== system test_ffts/r2_dit_fft/r2_dit_stage_1/r2_butterfly/ri_to_c ==
  re : Inport  Port=1  LatchInput=off
  im : Inport  Port=2  LatchInput=off
  concat : xbsIndex_r3/Concat  num_inputs=2  explicit_period=off  period=1  dbl_ovrd=off
  force_im : xbsIndex_r3/Reinterpret  force_arith_type=on  arith_type=Unsigned  force_bin_pt=on  bin_pt=0  force_valid=on
  force_re : xbsIndex_r3/Reinterpret  force_arith_type=on  arith_type=Unsigned  force_bin_pt=on  bin_pt=0  force_valid=on
  c : Outport
  wires:
  force_re/1 -> concat/1
  force_im/1 -> concat/2
  re/1 -> force_re/1
  concat/1 -> c/1
  im/1 -> force_im/1

== system test_ffts/r2_dit_fft/r2_dit_stage_1/r2_butterfly/ri_to_c1 ==
  re : Inport  Port=1  LatchInput=off
  im : Inport  Port=2  LatchInput=off
  concat : xbsIndex_r3/Concat  num_inputs=2  explicit_period=off  period=1  dbl_ovrd=off
  force_im : xbsIndex_r3/Reinterpret  force_arith_type=on  arith_type=Unsigned  force_bin_pt=on  bin_pt=0  force_valid=on
  force_re : xbsIndex_r3/Reinterpret  force_arith_type=on  arith_type=Unsigned  force_bin_pt=on  bin_pt=0  force_valid=on
  c : Outport
  wires:
  force_re/1 -> concat/1
  force_im/1 -> concat/2
  re/1 -> force_re/1
  concat/1 -> c/1
  im/1 -> force_im/1

== system test_ffts/r2_dit_fft/r2_dit_stage_2/biplex_commutator/delay_b ==
  in : Inport  Port=1  LatchInput=off
  slr : xbsIndex_r3/Delay  latency=16  reg_retiming=off  explicit_period=off  period=1  en=off  accept_only_valid=off  init_zero=on  dbl_ovrd=off  show_param=off
      settings: xl_area=[0, 0, 0, 0, 0, 0, 0]
  out : Outport
  wires:
  slr/1 -> out/1
  in/1 -> slr/1

== system test_ffts/r2_dit_fft/r2_dit_stage_2/biplex_commutator/delay_lo ==
  in : Inport  Port=1  LatchInput=off
  slr : xbsIndex_r3/Delay  latency=16  reg_retiming=off  explicit_period=off  period=1  en=off  accept_only_valid=off  init_zero=on  dbl_ovrd=off  show_param=off
      settings: xl_area=[0, 0, 0, 0, 0, 0, 0]
  out : Outport
  wires:
  slr/1 -> out/1
  in/1 -> slr/1

== system test_ffts/r2_dit_fft/r2_dit_stage_2/r2_butterfly/c_to_ri ==
  c : Inport  Port=1  LatchInput=off
  force_im : xbsIndex_r3/Reinterpret  force_arith_type=on  arith_type="Signed  (2's comp)"  force_bin_pt=on  bin_pt=0  force_valid=on
  force_re : xbsIndex_r3/Reinterpret  force_arith_type=on  arith_type="Signed  (2's comp)"  force_bin_pt=on  bin_pt=0  force_valid=on
  slice_im : xbsIndex_r3/Slice  mode=Lower Bit Location + Width  nbits=9  bit1=0  base1=MSB of Input  bit0=0  base0=LSB of Input  boolean_output=off  explicit_period=off  period=1  dbl_ovrd=off
  slice_re : xbsIndex_r3/Slice  mode=Upper Bit Location + Width  nbits=9  bit1=0  base1=MSB of Input  bit0=0  base0=LSB of Input  boolean_output=off  explicit_period=off  period=1  dbl_ovrd=off
  re : Outport
  im : Outport  Port=2
  wires:
  slice_re/1 -> force_re/1
  slice_im/1 -> force_im/1
  force_re/1 -> re/1
  force_im/1 -> im/1
  c/1 -> slice_re/1, slice_im/1

== system test_ffts/r2_dit_fft/r2_dit_stage_2/r2_butterfly/c_to_ri1 ==
  c : Inport  Port=1  LatchInput=off
  force_im : xbsIndex_r3/Reinterpret  force_arith_type=on  arith_type="Signed  (2's comp)"  force_bin_pt=on  bin_pt=0  force_valid=on
  force_re : xbsIndex_r3/Reinterpret  force_arith_type=on  arith_type="Signed  (2's comp)"  force_bin_pt=on  bin_pt=0  force_valid=on
  slice_im : xbsIndex_r3/Slice  mode=Lower Bit Location + Width  nbits=9  bit1=0  base1=MSB of Input  bit0=0  base0=LSB of Input  boolean_output=off  explicit_period=off  period=1  dbl_ovrd=off
  slice_re : xbsIndex_r3/Slice  mode=Upper Bit Location + Width  nbits=9  bit1=0  base1=MSB of Input  bit0=0  base0=LSB of Input  boolean_output=off  explicit_period=off  period=1  dbl_ovrd=off
  re : Outport
  im : Outport  Port=2
  wires:
  slice_re/1 -> force_re/1
  slice_im/1 -> force_im/1
  force_re/1 -> re/1
  force_im/1 -> im/1
  c/1 -> slice_re/1, slice_im/1
